simulink model "test08"  (R2021a)
settings: Solver=VariableStepAuto  StartTime=0.0  StopTime=tspan(end)  RelTol=1e-3
values from neighbouring files (symbols this model uses):
  crop_params = crop_p    [test08_script.m]
  scr_p = screen_p    [test08_script.m]
  x0_crop = crop_ic    [test08_script.m]
libraries: HORTISIM x14
(part 2 of 2)

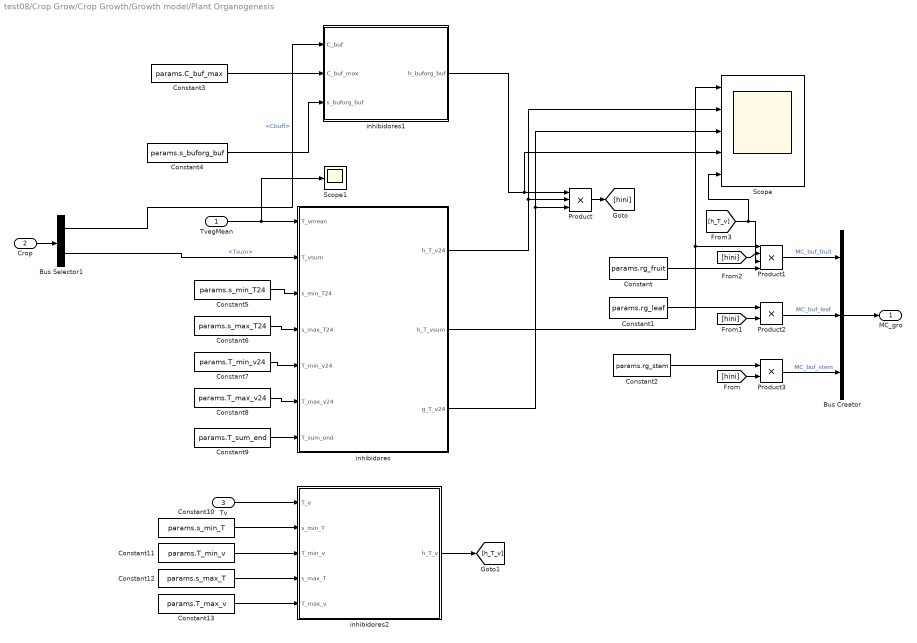
== system test08/Crop Grow/Crop Growth/Growth model/Plant Organogenesis  ==
  TvegMean : Inport
  Crop : Inport  Port=2
  Tv : Inport  Port=3
  Bus Creator : BusCreator  Inputs=3
  Bus Selector1 : BusSelector  OutputSignals=Carbon.Cbuff,Tsum
  Constant : Constant  Value=params.rg_fruit
  Constant1 : Constant  Value=params.rg_leaf
  Constant10 : Constant  Value=params.s_min_T
  Constant11 : Constant  Value=params.T_min_v
  Constant12 : Constant  Value=params.s_max_T
  Constant13 : Constant  Value=params.T_max_v
  Constant2 : Constant  Value=params.rg_stem
  Constant3 : Constant  Value=params.C_buf_max
  Constant4 : Constant  Value=params.s_buforg_buf
  Constant5 : Constant  Value=params.s_min_T24
  Constant6 : Constant  Value=params.s_max_T24
  Constant7 : Constant  Value=params.T_min_v24
  Constant8 : Constant  Value=params.T_max_v24
  Constant9 : Constant  Value=params.T_sum_end
  Product : Product  Inputs=3
  Product1 : Product  Inputs=4
  Product2 : Product
  Product3 : Product
  Scope : Scope  NumInputPorts=5
  Scope1 : Scope
  inhibidores : MATLAB Function  TreatAsAtomicUnit=on
  inhibidores1 : MATLAB Function  TreatAsAtomicUnit=on
  inhibidores2 : MATLAB Function  TreatAsAtomicUnit=on
  MC_gro : Outport
  wires:
  [h_T_v] -> Product1/3, Scope/5
  inhibidores2/1(h_T_v) -> [h_T_v]
  Constant13/1 -> inhibidores2/5(T_max_v)
  Constant12/1 -> inhibidores2/4(s_max_T)
  Constant11/1 -> inhibidores2/3(T_min_v)
  Constant10/1 -> inhibidores2/2(s_min_T)
  Tv/1 -> inhibidores2/1(T_v)
  Constant4/1 -> inhibidores1/3(s_buforg_buf)
  Bus Selector1/1 -> inhibidores1/1(C_buf)  "<Cbuff>"
  TvegMean/1 -> inhibidores/1(T_vmean), Scope1/1
  Bus Selector1/2 -> inhibidores/2(T_vsum)  "<Tsum>"
  Product3/1 -> Bus Creator/3  "MC_buf_stem"
  Product2/1 -> Bus Creator/2  "MC_buf_leaf"
  Product1/1 -> Bus Creator/1  "MC_buf_fruit"
  inhibidores/3(g_T_v24) -> Product/3, Scope/3
  inhibidores/1(h_T_v24) -> Product/2, Scope/2
  Bus Creator/1 -> MC_gro/1
  Crop/1 -> Bus Selector1/1
  Constant3/1 -> inhibidores1/2(C_buf_max)
  Constant5/1 -> inhibidores/3(s_min_T24)
  Constant6/1 -> inhibidores/4(s_max_T24)
  Constant7/1 -> inhibidores/5(T_min_v24)
  Constant8/1 -> inhibidores/6(T_max_v24)
  Constant9/1 -> inhibidores/7(T_sum_end)
  inhibidores1/1(h_buforg_buf) -> Product/1, Scope/4
  Constant/1 -> Product1/4
  inhibidores/2(h_T_vsum) -> Product1/1, Scope/1
  Constant1/1 -> Product2/1
  Constant2/1 -> Product3/1
  Product/1 -> [hini]
  [hini] -> Product3/2
  [hini] -> Product2/2
  [hini] -> Product1/2

== system test08/Crop Grow/Crop Growth/Growth model/Relative Growth ==
  Crop : Inport
  MC_leaf_prune : Inport  Port=2
  dCdt : Inport  Port=3
  harvest : Inport  Port=4
  Bus Selector : BusSelector  OutputSignals=Carbon.Cbuff,Carbon.Cfruit,Carbon.Cleaf,Relative.Rfruit,Relative.Rleaf,Relative.Rstem
  Bus Selector1 : BusSelector  OutputSignals=dC_fruit_dt,dC_fruit_dt,dC_fruit_dt
  Relative Growth : MATLAB Function  TreatAsAtomicUnit=on
  Vector Concatenate : Concatenate  NumInputs=3
  dRdt : Outport
  wires:
  harvest/1 -> Relative Growth/11(harvest)
  Bus Selector/1 -> Relative Growth/4(C_fruit)  "<Cbuff>"
  Bus Selector/2 -> Relative Growth/5(C_leaf)  "<Cfruit>"
  Bus Selector/3 -> Relative Growth/6(C_stem)  "<Cleaf>"
  Bus Selector/4 -> Relative Growth/7(R_fruit)  "<Rfruit>"
  Bus Selector/5 -> Relative Growth/8(R_leaf)  "<Rleaf>"
  Bus Selector/6 -> Relative Growth/9(R_stem)  "<Rstem>"
  Bus Selector1/3 -> Relative Growth/3(dC_stem_dt)  "<dC_fruit_dt>"
  Bus Selector1/1 -> Relative Growth/1(dC_fruit_dt)  "<dC_fruit_dt>"
  Bus Selector1/2 -> Relative Growth/2(dC_leaf_dt)  "<dC_fruit_dt>"
  dCdt/1 -> Bus Selector1/1
  Crop/1 -> Bus Selector/1
  Vector Concatenate/1 -> dRdt/1
  MC_leaf_prune/1 -> Relative Growth/10(MC_leaf_prune)
  Relative Growth/1(dR_fruit_dt) -> Vector Concatenate/1
  Relative Growth/3(dR_stem_dt) -> Vector Concatenate/3
  Relative Growth/2(dR_leaf_dt) -> Vector Concatenate/2

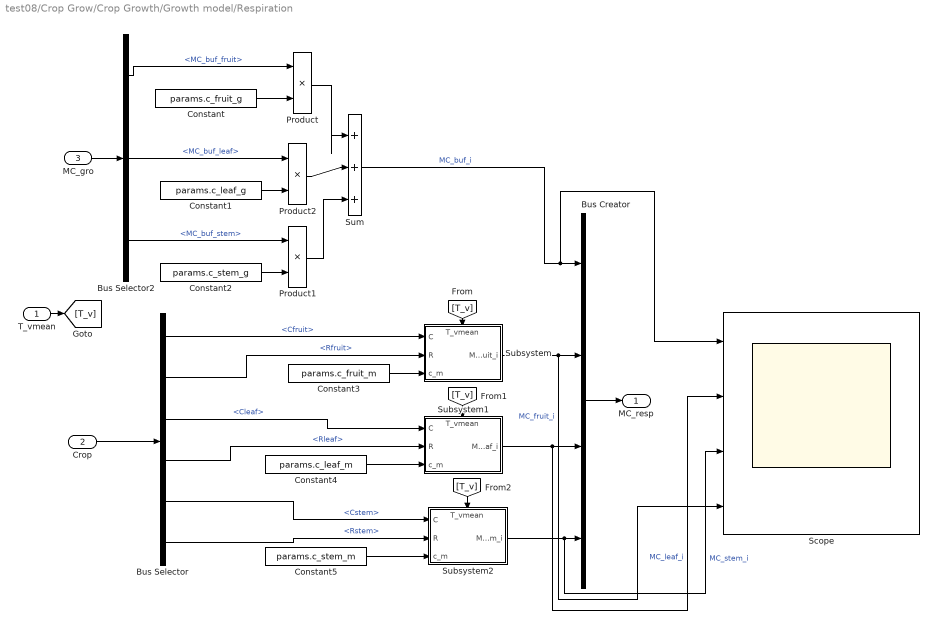
== system test08/Crop Grow/Crop Growth/Growth model/Respiration ==
  T_vmean : Inport
  Crop : Inport  Port=2
  MC_gro : Inport  Port=3
  Bus Creator : BusCreator  Inputs=4
  Bus Selector : BusSelector  OutputSignals=Carbon.Cfruit,Relative.Rfruit,Carbon.Cleaf,Relative.Rleaf,Carbon.Cstem,Relative.Rstem
  Bus Selector2 : BusSelector  OutputSignals=MC_buf_fruit,MC_buf_leaf,MC_buf_stem
  Constant : Constant  Value=params.c_fruit_g
  Constant1 : Constant  Value=params.c_leaf_g
  Constant2 : Constant  Value=params.c_stem_g
  Constant3 : Constant  Value=params.c_fruit_m
  Constant4 : Constant  Value=params.c_leaf_m
  Constant5 : Constant  Value=params.c_stem_m
  Product : Product
  Product1 : Product
  Product2 : Product
  Scope : Scope  NumInputPorts=4
  Subsystem : Subsystem
      settings: PortSchema="{\"entries\":[{\"content\":{\"sides\":[{\"content\":{\"connectorIds\":[\"In1\",\"In2\",\"In3\"]},\"type\":\"ConnectorPlacement.EquallySpacedRectSide\",\"uuid\":\"e383cf86-92c2-4a3a-a03f-0f03c9e6b06e\"},{\"content\":{\"connectorIds\":[\"Out1\"],\"side\":\"RIGHT\"},\"type\":\"ConnectorPlacement.EquallySpacedRectSide\",\"uuid\":\"c4c6234d-4969-4652-ba5e-e62d60415ae5\"},{\"content\":{\"connectorIds\":[\"In4\"],\"side\":\"TOP\"},\"type\":\"ConnectorPlacement.EquallySpacedRectSide\",\"uuid\":\"e372fef3-870c-4656-925c-98a7f16866f7\"}]},\"type\":\"ConnectorPlacement.EquallySpacedConnector\",\"uuid\":\"336e0ef1-3fb5-46ea-bbca-17f64dad2455\"}],\"packageUris\":[\"http://schema.mathworks.com/mf0/Connector/R2020b\"],\"version\":\"1.0\"}"
  Subsystem1 : Subsystem
      settings: PortSchema="{\"entries\":[{\"content\":{\"sides\":[{\"content\":{\"connectorIds\":[\"In1\",\"In2\",\"In3\"]},\"type\":\"ConnectorPlacement.EquallySpacedRectSide\",\"uuid\":\"e383cf86-92c2-4a3a-a03f-0f03c9e6b06e\"},{\"content\":{\"connectorIds\":[\"Out1\"],\"side\":\"RIGHT\"},\"type\":\"ConnectorPlacement.EquallySpacedRectSide\",\"uuid\":\"c4c6234d-4969-4652-ba5e-e62d60415ae5\"},{\"content\":{\"connectorIds\":[\"In4\"],\"side\":\"TOP\"},\"type\":\"ConnectorPlacement.EquallySpacedRectSide\",\"uuid\":\"e372fef3-870c-4656-925c-98a7f16866f7\"}]},\"type\":\"ConnectorPlacement.EquallySpacedConnector\",\"uuid\":\"336e0ef1-3fb5-46ea-bbca-17f64dad2455\"}],\"packageUris\":[\"http://schema.mathworks.com/mf0/Connector/R2020b\"],\"version\":\"1.0\"}"
  Subsystem2 : Subsystem
      settings: PortSchema="{\"entries\":[{\"content\":{\"sides\":[{\"content\":{\"connectorIds\":[\"In1\",\"In2\",\"In3\"]},\"type\":\"ConnectorPlacement.EquallySpacedRectSide\",\"uuid\":\"e383cf86-92c2-4a3a-a03f-0f03c9e6b06e\"},{\"content\":{\"connectorIds\":[\"Out1\"],\"side\":\"RIGHT\"},\"type\":\"ConnectorPlacement.EquallySpacedRectSide\",\"uuid\":\"c4c6234d-4969-4652-ba5e-e62d60415ae5\"},{\"content\":{\"connectorIds\":[\"In4\"],\"side\":\"TOP\"},\"type\":\"ConnectorPlacement.EquallySpacedRectSide\",\"uuid\":\"e372fef3-870c-4656-925c-98a7f16866f7\"}]},\"type\":\"ConnectorPlacement.EquallySpacedConnector\",\"uuid\":\"336e0ef1-3fb5-46ea-bbca-17f64dad2455\"}],\"packageUris\":[\"http://schema.mathworks.com/mf0/Connector/R2020b\"],\"version\":\"1.0\"}"
  Sum : Sum  Inputs=|+++
  MC_resp : Outport
  wires:
  Bus Selector/6 -> Subsystem2/2(R)  "<Rstem>"
  Bus Selector/5 -> Subsystem2/1(C)  "<Cstem>"
  Bus Selector/4 -> Subsystem1/2(R)  "<Rleaf>"
  Bus Selector/3 -> Subsystem1/1(C)  "<Cleaf>"
  Bus Selector/2 -> Subsystem/2(R)  "<Rfruit>"
  Bus Selector/1 -> Subsystem/1(C)  "<Cfruit>"
  Crop/1 -> Bus Selector/1
  MC_gro/1 -> Bus Selector2/1
  Subsystem2/1(MC_steam_i) -> Bus Creator/4, Scope/3  "MC_stem_i"
  Subsystem1/1(MC_leaf_i) -> Bus Creator/3, Scope/2  "MC_leaf_i"
  Subsystem/1(MC_fruit_i) -> Bus Creator/2, Scope/4  "MC_fruit_i"
  Bus Creator/1 -> MC_resp/1
  Bus Selector2/1 -> Product/1  "<MC_buf_fruit>"
  Bus Selector2/2 -> Product2/1  "<MC_buf_leaf>"
  Bus Selector2/3 -> Product1/1  "<MC_buf_stem>"
  Sum/1 -> Bus Creator/1, Scope/1  "MC_buf_i"
  Product/1 -> Sum/1
  Constant2/1 -> Product1/2
  Constant/1 -> Product/2
  Constant1/1 -> Product2/2
  Product2/1 -> Sum/2
  Product1/1 -> Sum/3
  T_vmean/1 -> [T_v]
  Constant3/1 -> Subsystem/3(c_m)
  [T_v] -> Subsystem/4(T_vmean)
  [T_v] -> Subsystem1/4(T_vmean)
  [T_v] -> Subsystem2/4(T_vmean)
  Constant4/1 -> Subsystem1/3(c_m)
  Constant5/1 -> Subsystem2/3(c_m)

== system test08/Crop Grow/Crop Growth/Growth model/Subsystem2 ==
  " " : Inport
  "         " : Inport  Port=2
  Bus Creator : BusCreator  Inputs=5
  Demux : Demux
  "   " : Outport
  wires:
  Demux/4 -> Bus Creator/5  "MC_stem_i"
  Bus Creator/1 -> "   "/1
  " "/1 -> Bus Creator/1  "MC_i_buf"
  Demux/3 -> Bus Creator/4  "MC_leaf_i"
  Demux/1 -> Bus Creator/2  "MC_buf_i"
  Demux/2 -> Bus Creator/3  "MC_fruit_i"
  "         "/1 -> Demux/1

== system test08/Crop Grow/Merges/Subsystem/Convertion Ratio ==
  Constant : Constant
  Constant1 : Constant  Value=params.fraction_DM
  Divide : Product  Inputs=*/
  Minus : Sum  Inputs=+-
  Out1 : Outport
  wires:
  Divide/1 -> Minus/1
  Constant/1 -> Minus/2, Divide/1
  Constant1/1 -> Divide/2
  Minus/1 -> Out1/1

== system test08/Ferrtirrigation Controler/Irrigation Controler/If Action Subsystem/If Action Subsystem ==
  Action Port : ActionPort  ActionPortLabel=if(u1 > 0.5)
  Constant : Constant  Value=0
  Out1 : Outport
  wires:
  Constant/1 -> Out1/1

== system test08/Ferrtirrigation Controler/Irrigation Controler/If Action Subsystem/If Action Subsystem1 ==
  Action Port : ActionPort  ActionPortLabel=else
  Constant : Constant
  Out1 : Outport
  wires:
  Constant/1 -> Out1/1

== system test08/Subsystem/Screen Controler/Subsystem/If Action Subsystem ==
  Action Port : ActionPort  ActionPortLabel=if(u1 < 10)
  Constant : Constant  Value=100
  Out1 : Outport
  wires:
  Constant/1 -> Out1/1

== system test08/Subsystem/Screen Controler/Subsystem/If Action Subsystem1 ==
  EC : Inport
  Action Port : ActionPort  ActionPortLabel=else
  Constant : Constant  Value=params.Radthreshold
  Gain1 : Gain  Gain=100
  Minus1 : Sum  Inputs=+-
  "Theta " : Subsystem
  Out1 : Outport
  wires:
  Constant/1 -> Minus1/2
  "Theta "/1(Out1) -> Gain1/1
  Minus1/1 -> "Theta "/1(In1)
  EC/1 -> Minus1/1
  Gain1/1 -> Out1/1

== system test08/Subsystem/Screen Controler/Subsystem/Smooth Rad ==
  In1 : Inport
  Gain : Gain  Gain=10
  Integrator1 : Integrator
  Minus2 : Sum  Inputs=+-
  Sec2Days1 : Gain  Gain=24*3600
  Out1 : Outport
  wires:
  In1/1 -> Minus2/1
  Sec2Days1/1 -> Integrator1/1
  Integrator1/1 -> Out1/1, Minus2/2
  Minus2/1 -> Gain/1
  Gain/1 -> Sec2Days1/1

== system test08/Crop Grow/Crop Growth/Growth model/Respiration/Subsystem ==
  C : Inport
  R : Inport  Port=2
  c_m : Inport  Port=3
  T_vmean : Inport  Port=4
  Exponetial Term : Subsystem
  Gain : Gain  Gain=0.1
  Minus : Sum  Inputs=+-
  Power : Math  Operator=pow  SaturateOnIntegerOverflow=on
  Product2 : Product  Inputs=4
  Q_10 : Constant  Value=2
  T_25 : Constant  Value=298.1500
  MC_fruit_i : Outport
  wires:
  T_vmean/1 -> Minus/1
  T_25/1 -> Minus/2
  Minus/1 -> Gain/1
  Gain/1 -> Power/2
  R/1 -> Exponetial Term/1(In1)
  Exponetial Term/1(Out1) -> Product2/1
  Q_10/1 -> Power/1
  Power/1 -> Product2/2
  c_m/1 -> Product2/3
  C/1 -> Product2/4
  Product2/1 -> MC_fruit_i/1

== system test08/Crop Grow/Crop Growth/Growth model/Respiration/Subsystem1 ==
  C : Inport
  R : Inport  Port=2
  c_m : Inport  Port=3
  T_vmean : Inport  Port=4
  Exponetial Term : Subsystem
  Gain : Gain  Gain=0.1
  Minus : Sum  Inputs=+-
  Power : Math  Operator=pow  SaturateOnIntegerOverflow=on
  Product2 : Product  Inputs=4
  Q_10 : Constant  Value=2
  T_25 : Constant  Value=298.1500
  MC_leaf_i : Outport
  wires:
  T_vmean/1 -> Minus/1
  T_25/1 -> Minus/2
  Minus/1 -> Gain/1
  Gain/1 -> Power/2
  R/1 -> Exponetial Term/1(In1)
  Exponetial Term/1(Out1) -> Product2/1
  Q_10/1 -> Power/1
  Power/1 -> Product2/2
  c_m/1 -> Product2/3
  C/1 -> Product2/4
  Product2/1 -> MC_leaf_i/1

== system test08/Crop Grow/Crop Growth/Growth model/Respiration/Subsystem2 ==
  C : Inport
  R : Inport  Port=2
  c_m : Inport  Port=3
  T_vmean : Inport  Port=4
  Exponetial Term : Subsystem
  Gain : Gain  Gain=0.1
  Minus : Sum  Inputs=+-
  Power : Math  Operator=pow  SaturateOnIntegerOverflow=on
  Product2 : Product  Inputs=4
  Q_10 : Constant  Value=2
  T_25 : Constant  Value=298.1500
  MC_steam_i : Outport
  wires:
  T_vmean/1 -> Minus/1
  T_25/1 -> Minus/2
  Minus/1 -> Gain/1
  Gain/1 -> Power/2
  R/1 -> Exponetial Term/1(In1)
  Exponetial Term/1(Out1) -> Product2/1
  Q_10/1 -> Power/1
  Power/1 -> Product2/2
  c_m/1 -> Product2/3
  C/1 -> Product2/4
  Product2/1 -> MC_steam_i/1

== system test08/Subsystem/Screen Controler/Subsystem/If Action Subsystem1/Theta  ==
  In1 : Inport
  Constant1 : Constant  Value=0.5
  Gain : Gain  Gain=0.5
  Sign : Signum  ZeroCross=off
  Sum : Sum  Inputs=|++
  Out1 : Outport
  wires:
  Sign/1 -> Gain/1
  Sum/1 -> Out1/1
  Gain/1 -> Sum/1
  In1/1 -> Sign/1
  Constant1/1 -> Sum/2

== system test08/Crop Grow/Crop Growth/Growth model/Respiration/Subsystem/Exponetial Term ==
  In1 : Inport
  Constant : Constant
  Exp : Math  SaturateOnIntegerOverflow=on
  Gain1 : Gain  Gain=-1
  Minus1 : Sum  Inputs=+-
  Product1 : Product
  regression coefficient in maintenance respiration function [s] : Constant  Value=2850000
  Out1 : Outport
  wires:
  In1/1 -> Product1/1
  Minus1/1 -> Out1/1
  regression coefficient in maintenance respiration function [s]/1 -> Product1/2
  Exp/1 -> Minus1/2
  Gain1/1 -> Exp/1
  Constant/1 -> Minus1/1
  Product1/1 -> Gain1/1

== system test08/Crop Grow/Crop Growth/Growth model/Respiration/Subsystem1/Exponetial Term ==
  In1 : Inport
  Constant : Constant
  Exp : Math  SaturateOnIntegerOverflow=on
  Gain1 : Gain  Gain=-1
  Minus1 : Sum  Inputs=+-
  Product1 : Product
  regression coefficient in maintenance respiration function [s] : Constant  Value=2850000
  Out1 : Outport
  wires:
  In1/1 -> Product1/1
  Minus1/1 -> Out1/1
  regression coefficient in maintenance respiration function [s]/1 -> Product1/2
  Exp/1 -> Minus1/2
  Gain1/1 -> Exp/1
  Constant/1 -> Minus1/1
  Product1/1 -> Gain1/1

== system test08/Crop Grow/Crop Growth/Growth model/Respiration/Subsystem2/Exponetial Term ==
  In1 : Inport
  Constant : Constant
  Exp : Math  SaturateOnIntegerOverflow=on
  Gain1 : Gain  Gain=-1
  Minus1 : Sum  Inputs=+-
  Product1 : Product
  regression coefficient in maintenance respiration function [s] : Constant  Value=2850000
  Out1 : Outport
  wires:
  In1/1 -> Product1/1
  Minus1/1 -> Out1/1
  regression coefficient in maintenance respiration function [s]/1 -> Product1/2
  Exp/1 -> Minus1/2
  Gain1/1 -> Exp/1
  Constant/1 -> Minus1/1
  Product1/1 -> Gain1/1

== matlab function test08/Crop Grow/Crop Growth/Growth model/Photosynthesis/MATLAB Function ==
  data: T_v input; LAI input; Gamma output
function Gamma = fcn(T_v,LAI)

T_k = 273.1500; % zero celsius [K]
c_Gamma         = 1.7000e-06; % effect of canopy temperature on CO2 compensation point [mol{CO2}/mol{air}/K]

Gamma = (c_Gamma*(T_v - T_k)./LAI + 20*c_Gamma*(1 - 1./LAI)); % The CO2 compensation point [mol{CO2}/mol{air}]

== matlab function test08/Crop Grow/Crop Growth/Growth model/Photosynthesis/Photosyntesis ==
  data: QS_v_VIS input; MC_i_buf output; LAI input; C_c input; rho_i input; T_v input; Gamma input; A_v input; PAR output; P output; Resp output; C_stom output
   function [MC_i_buf,PAR,P,Resp,C_stom] = fcn(QS_v_VIS,LAI,C_c,rho_i,T_v,Gamma,A_v)

%%
% CONSTANTS
% =========
N_A =    6.0221e+23; % Avogadro's number
M_a = 0.0290; % molar mass of dry air [kg/mol]                                                                 
R =     8.3140; % gas constant [J/mol/K]
M_c = 0.0440; % molar mass of CO2 [kg/mol]
T_25 = 298.1500; % K
%
% PHOTOSYNTHESIS MODEL - VANTHOOR
% ===============================
J_max_25        = 2.1000e-04; % maximum rate of electron transport at 25 C [mol{e}/m^2{leaf}/s]
alph            = 0.3850; % conversion factor from photons to electrons [mol{e}/mol{phot}]
theta_constant  = 0.7000; % degree of curvature of the electron transport rate [-]
S               = 710; % entropy term for J_pot calculation [J/mol/K]
HH              = 220000; % deactivation energy for J_pot calculation [J/mol]
E_j             = 37000; % activation energy for J_pot calculation [J/mol]
heat_phot       = 3.6368e-19; % conversion rate from incident energy to number of photons [num{photons}/J]
eta             = 0.6700; % conversion factor from CO2 in the air to CO2 in the stomata [-]
M_carb          = 0.0300; % molar mass of CH2O [kg/mol]

%%

PAR = QS_v_VIS/heat_phot/N_A./A_v; 
% The number of moles of photosynthetically active photons per unit area of planted floor [mol{phot}/m^2/s]
%J/s/(J/photon)/(photons/mol)/m^2 cf Vanthoor 2.3mumol(photons)/J

C_c_molar=(C_c./rho_i).*(M_a/M_c);

%C_stom = eta*C_c_molar; % Stomatal CO2 concentration [mol{CO2}/mol{air}] 
C_stom = eta*C_c_molar; % Stomatal CO2 concentration [mol{CO2}/mol{air}] 

J_pot = LAI*J_max_25.*exp(E_j*(T_v - T_25)./(R*T_v*T_25)).*...
    (1 + exp((S*T_25 - HH)/(R*T_25)))./(1 + exp((S*T_v - HH)./(R*T_v))); % [mol{e}/m^2{floor}s]
%
J = (J_pot + alph*PAR - sqrt((J_pot + alph*PAR).^2 - 4*theta_constant*J_pot*alph.*PAR))/(2*theta_constant);
%
P = J.*(C_stom - Gamma)./(4*(C_stom + 2*Gamma)); % Photosynthesis rate [mol{CO2}/s]
%
Resp = P.*Gamma./C_stom; % Photorespiration rate
%
MC_i_buf = (M_carb.*(P - Resp)); % The net photosynthesis rate [kg{CH2O}/m^2/s]

== matlab function test08/Crop Grow/Crop Growth/Growth model/Plant Organogenesis /inhibidores ==
  data: T_vmean input; T_vsum input; s_min_T24 input; s_max_T24 input; T_min_v24 input; T_max_v24 input; h_T_v24 output; h_T_vsum output; g_T_v24 output; T_sum_end input
function [h_T_v24,h_T_vsum,g_T_v24] = growth_diff(T_vmean,T_vsum,s_min_T24,s_max_T24,T_min_v24,T_max_v24,T_sum_end)



T_k = 273.15; % zero celsius [K]
%h_T_v24 = 1./(1 + exp(s_min_T24*((T_vmean-T_k) - T_min_v24)))./(1 + exp(s_max_T24*((T_vmean-T_k) - T_max_v24))); 

%k = 0.02;
%h_T_vsum = 0.5 + 0.5*tanh(k*(T_vsum - T_v_start_fruit));

g_T_v24 = 0.047*(T_vmean - T_k) + 0.06;




h_T_v24 = 1./(1 + exp(s_min_T24*((T_vmean-T_k) - T_min_v24)))./(1 + exp(s_max_T24*((T_vmean-T_k) - T_max_v24))); 

h_T_vsum = 0.5*(T_vsum./T_sum_end + sqrt((T_vsum./T_sum_end).^2 + 1e-4)) ...
    - 0.5*(((T_vsum - T_sum_end)/T_sum_end)+sqrt(((T_vsum - T_sum_end)/T_sum_end).^2 + 1e-4)); 


end

== matlab function test08/Crop Grow/Crop Growth/Growth model/Plant Organogenesis /inhibidores1 ==
  data: C_buf input; h_buforg_buf output; C_buf_max input; s_buforg_buf input
function h_buforg_buf  = growth_diff(C_buf,C_buf_max,s_buforg_buf)

%C_buf_min = 0.05*C_buf_max;  
%
%x = (C_buf - C_buf_min);
%h_buforg_buf = (x>0)*(1-exp(-x/0.005));

C_buf_min = 0.05*C_buf_max;
h_buforg_buf =1./(1 + exp(s_buforg_buf*(C_buf - C_buf_min)));


end

== matlab function test08/Crop Grow/Crop Growth/Growth model/Relative Growth/Relative Growth ==
  data: dC_fruit_dt input; dC_leaf_dt input; dC_stem_dt input; C_fruit input; C_leaf input; C_stem input; R_fruit input; R_leaf input; R_stem input; dR_fruit_dt output; dR_leaf_dt output; dR_stem_dt output; MC_leaf_prune input; harvest input
function [dR_fruit_dt,dR_leaf_dt,dR_stem_dt] = fcn(dC_fruit_dt,dC_leaf_dt,dC_stem_dt,C_fruit,C_leaf,C_stem,R_fruit,R_leaf,R_stem,MC_leaf_prune, harvest)



% Plant growth
dR_fruit_dt = ((dC_fruit_dt + harvest)./C_fruit - R_fruit);
dR_leaf_dt = ((dC_leaf_dt + MC_leaf_prune)./C_leaf - R_leaf);
dR_stem_dt = (dC_stem_dt./C_stem - R_stem);

== matlab function test08/Crop Grow/Transpiration/MATLAB Function1 ==
  data: vpd input; T_v input; HV input; QS_int input; rho_i input; hL_v_i output
function hL_v_i  = fcn(  vpd,T_v,HV,QS_int ,rho_i )

%%
% CONSTANTS
% =========
T_k  =  273.1500;   % zero celsius [K]
c_i  =  1.0032e+03; % heat capacity of humid air [J/kg/K]                        
H_fg =  2437000;    % latent heat of condensation of water [J/kg]
Le   =  0.8190;     % Lewis number [-] 

% VEGETATION CHARACTERISTICS
%%
Heavy_vpd = vpd/1000 < 0.8;
r_i_vpd   = Heavy_vpd.*(1 + 4.3*(vpd/1000).^2) + (1 - Heavy_vpd)*3.8;

r_st      = 82*((QS_int + 4.3)./(QS_int + 0.54)).*(1 + 0.023*(T_v - T_k - 24.5).^2).*r_i_vpd; %[s/m]

hL_v_i = 2*H_fg./(rho_i*c_i).*(Le^(2/3)./HV + r_st./(rho_i*c_i)).^(-1); %

== matlab function test08/Crop Grow/Crop Growth/Growth model/Plant Organogenesis /inhibidores2 ==
  data: T_v input; s_min_T input; T_min_v input; s_max_T input; T_max_v input; h_T_v output
function h_T_v = growth_diff(T_v,s_min_T,T_min_v,s_max_T,T_max_v)



T_k = 273.15; % zero celsius [K]


h_T_v = 1./(1 + exp(s_min_T*((T_v-T_k) - T_min_v)))./(1 + exp(s_max_T*((T_v-T_k) - T_max_v))); 

end

== matlab function test08/Crop Grow/Air Convection/ Temperature ==
  data: QS_v_VIS input; QT_v_i input; QV_v_i input; dT_v_dt output; A_v input; LAI input; msd_v input
function dT_v_dt  = fcn(QS_v_VIS,QT_v_i,QV_v_i,A_v,LAI,msd_v)

c_v   = 4180; % heat capacity of vegetation [J/kgK]
%msd_v = p.msd_v; % surface density [kg/m^2]
%A_v   = p.A_v;

%% Vegetation Temperature
c_Tv = 1./(c_v* A_v.*LAI.*msd_v);
% 
dT_v_dt = c_Tv*( - QV_v_i  - QT_v_i + QS_v_VIS); 
%% Air Temperature

== matlab function test08/Crop Grow/Air Convection/Subsystem/Convection1 ==
  data: T_i input; Nu input; T_v input; LAI input; QV_v_i output; A_v input; HV output; d_v input
function [QV_v_i,HV] = fcn(T_i,Nu,T_v,LAI,A_v,d_v)


lambda = 0.250; % thermal conductivity of air [W/m/K]
A_v_exp = LAI*A_v; % Area vegetation exposed
QV_v_i = A_v_exp.*Nu*lambda.*(T_v - T_i)/d_v;
HV = Nu*lambda/d_v; % Used in the transpiration term

== matlab function test08/Crop Grow/Air Convection/Subsystem/Raynols ==
  data: Nu output; T_i input; T_v input; d_v input; int_air_speed input
 function Nu  = fcn(T_i,T_v,d_v,int_air_speed )


% CONSTANTS
% =========
g =     9.8100; % acceleration due to gravity [m/s^2]
nu = 1.5100e-05; % kinematic viscosity [m^2/s]
% VEGETATION CHARACTERISTICS
% ==========================
%d_v = p.d_v; % characteristic leaf length [m]
%int_air_speed = p.int_air_speed;
%%

%%      Convection
% Vegetation to internal air
Gr = g*d_v^3./(T_i*nu^2).*abs(T_v - T_i);
Re = int_air_speed*d_v/nu;
Nu = lamorturb(Gr, Re);

== matlab function test08/Crop Grow/Crop Growth/Growth model/Growth Organs/Derivatives ==
  data: MC_i_buf input; dC_buff_dt output; dC_fruit_dt output; dC_leaf_dt output; dC_stem_dt output; MC_buf_fruit input; MC_buf_leaf input; MC_buf_stem input; MC_buff_i input; MC_fruit_i input; MC_leaf_i input; MC_stem_i input; MC_leaf_prune input; harvest input
function [dC_buff_dt,dC_fruit_dt,dC_leaf_dt,dC_stem_dt] = fcn(MC_i_buf,MC_buf_fruit,MC_buf_leaf,MC_buf_stem,MC_buff_i,MC_fruit_i,MC_leaf_i,MC_stem_i,MC_leaf_prune, harvest)
%% CALCULATING DERIVATIVES


dC_buff_dt = MC_i_buf - MC_buf_fruit - MC_buf_leaf - MC_buf_stem - MC_buff_i ;

% Plant carbon exchange
dC_fruit_dt = MC_buf_fruit - MC_fruit_i - harvest;

dC_leaf_dt  = MC_buf_leaf  - MC_leaf_i - MC_leaf_prune;

dC_stem_dt  = MC_buf_stem  - MC_stem_i ;
